simulink model "Model_3"  (R2019b)
settings: Solver=ode15s  StartTime=0.0  StopTime=35  MaxStep=0.005  RelTol=1e-3
model workspace (MATLAB code in the model file):
  | ms = 135;
  | mf = 5;
  | mr = 10;
  | m = ms + (mf + mr);
  | a = 0.7;
  | b = 0.7;
  | Cd = 0.8;
  | Af = 1;
  | h_cg = 0.5;
  | kf = 10000;
  | kr = 15000;
  | cf = 5000;
  | cr = 5000;
  | I = 500;
  | kt = 175000;
values from neighbouring files (symbols this model uses):
  GR = 6.5    [Model_1_timeto40.m]    (also in Model_1_timeto60.m; Model_3_topspeed.m)
  Pmax = P(i,j)    [Model_1_timeto40.m]    (also in Model_1_timeto60.m; Model_3_topspeed.m = P(i))
libraries: autolibshared x2
(part 3 of 3)

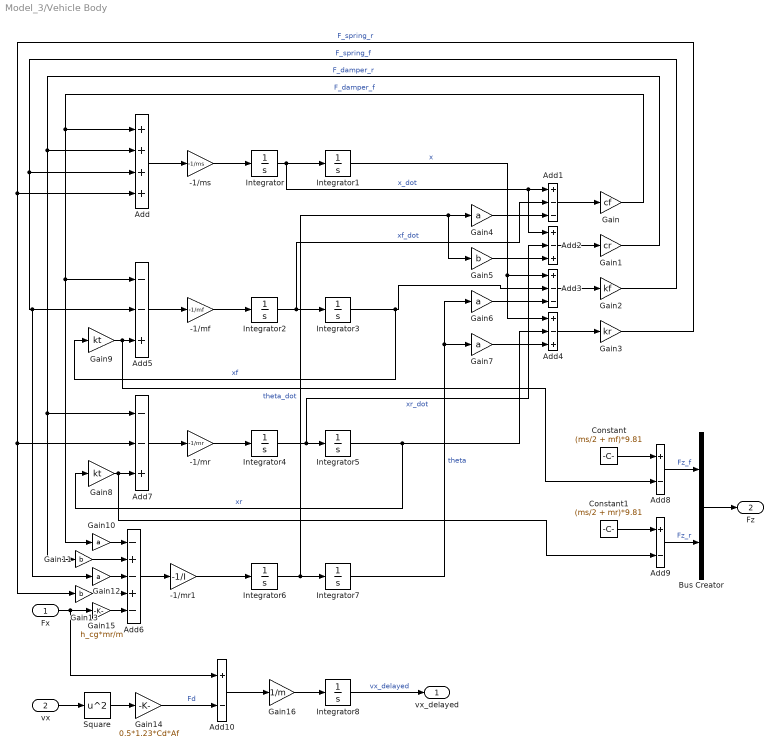
== system Model_3/Vehicle Body ==
  Fx : Inport
  vx : Inport  Port=2
  -1/mf : Gain  Gain=-1/mf
  -1/mr : Gain  Gain=-1/mr
  -1/mr1 : Gain  Gain=-1/I
  -1/ms : Gain  Gain=-1/ms
  Add : Sum  Inputs=++++
  Add1 : Sum  Inputs=+--
  Add10 : Sum  Inputs=+-
  Add2 : Sum  Inputs=+-+
  Add3 : Sum  Inputs=+--
  Add4 : Sum  Inputs=+-+
  Add5 : Sum  Inputs=--+
  Add6 : Sum  Inputs=-+-+-
  Add7 : Sum  Inputs=--+
  Add8 : Sum  Inputs=+-
  Add9 : Sum  Inputs=+-
  Bus Creator : BusCreator  Inputs=2
  Constant : Constant  Value=(ms/2 + mf)*9.81
  Constant1 : Constant  Value=(ms/2 + mr)*9.81
  Gain : Gain  Gain=cf
  Gain1 : Gain  Gain=cr
  Gain{4,6..7,10,12} (5 alike) : Gain  Gain=a
  Gain11 : Gain  Gain=b
  Gain13 : Gain  Gain=b
  Gain14 : Gain  Gain=0.5*1.23*Cd*Af
  Gain15 : Gain  Gain=h_cg*mr/m
  Gain16 : Gain  Gain=1/m
  Gain2 : Gain  Gain=kf
  Gain3 : Gain  Gain=kr
  Gain5 : Gain  Gain=b
  Gain8 : Gain  Gain=kt
  Gain9 : Gain  Gain=kt
  Integrator{,1..8} (9 alike) : Integrator
  Square : Math  Operator=square  SignedPower=off  SaturateOnIntegerOverflow=on
  vx_delayed : Outport
  Fz : Outport  Port=2
  wires:
  Integrator1/1 -> Add4/1, Add3/1  "x"
  Integrator/1 -> Integrator1/1, Add2/1, Add1/1  "x_dot"
  -1/ms/1 -> Integrator/1
  Add/1 -> -1/ms/1
  Gain/1 -> Gain10/1, Add5/1, Add/1  "F_damper_f"
  Gain3/1 -> Gain13/1, Add7/2, Add/4  "F_spring_r"
  Gain2/1 -> Gain12/1, Add5/2, Add/3  "F_spring_f"
  Gain1/1 -> Gain11/1, Add7/1, Add/2  "F_damper_r"
  Add1/1 -> Gain/1
  Add2/1 -> Gain1/1
  Add3/1 -> Gain2/1
  Add4/1 -> Gain3/1
  -1/mf/1 -> Integrator2/1
  Integrator2/1 -> Add1/2, Integrator3/1  "xf_dot"
  Integrator3/1 -> Gain9/1, Add3/2  "xf"
  Integrator5/1 -> Gain8/1, Add4/2  "xr"
  Integrator4/1 -> Add2/2, Integrator5/1  "xr_dot"
  -1/mr/1 -> Integrator4/1
  -1/mr1/1 -> Integrator6/1
  Integrator6/1 -> Gain5/1, Gain4/1, Integrator7/1  "theta_dot"
  Integrator7/1 -> Gain7/1, Gain6/1  "theta"
  Gain4/1 -> Add1/3
  Gain5/1 -> Add2/3
  Gain6/1 -> Add3/3
  Gain7/1 -> Add4/3
  Add5/1 -> -1/mf/1
  Add7/1 -> -1/mr/1
  Add6/1 -> -1/mr1/1
  Gain8/1 -> Add7/3, Add9/2
  Gain9/1 -> Add8/2, Add5/3
  Gain10/1 -> Add6/1
  Gain11/1 -> Add6/2
  Gain12/1 -> Add6/3
  Gain13/1 -> Add6/4
  Fx/1 -> Add10/1, Gain15/1
  Gain15/1 -> Add6/5
  vx/1 -> Square/1
  Constant/1 -> Add8/1
  Add8/1 -> Bus Creator/1  "Fz_f"
  Constant1/1 -> Add9/1
  Add9/1 -> Bus Creator/2  "Fz_r"
  Bus Creator/1 -> Fz/1
  Square/1 -> Gain14/1
  Gain14/1 -> Add10/2  "Fd"
  Add10/1 -> Gain16/1
  Gain16/1 -> Integrator8/1
  Integrator8/1 -> vx_delayed/1  "vx_delayed"
